simulink library "RespiratorCtrlLib"  (R2018b)
settings: Solver=VariableStepAuto  StartTime=0.0  StopTime=10.0  RelTol=1e-3
undefined symbols (not defined in the file or in its folder): AnalogMax, AnalogMin, aValveFullClose, aValveFullOpen, aValvePwm100, eSupervisorStates, fpDiffQAirInhalation, fpStatQAirInhalation, pDiffQAirAutoOffsetMax, pDiffQAirAutoOffsetMin, pDiffQAirAutoOffsetRateMax, pDiffQAirInhalationOffset, pDiffQAirScaledMax, pDiffQAirScaledMin, PressureMax, PressureMin, pStatQAirAutoOffsetMax, pStatQAirAutoOffsetMin, pStatQAirAutoOffsetRateMax, pStatQAirInhalationOffset, pStatQAirScaledMax, pStatQAirScaledMin, rPwmZeroDeg, VAnalogInputSpan, VpDiffQAirAnalogicDiagMax, VpDiffQAirAnalogicDiagMin, VpDiffQAirAnalogicMax, VpDiffQAirAnalogicMin, VpStatQAirAnalogicDiagMax, VpStatQAirAnalogicDiagMin, VpStatQAirAnalogicMax, VpStatQAirAnalogicMin
libraries: simulink x16, mbedblockslib x4, simulink_extras x2, $bdroot x2
(part 2 of 2)

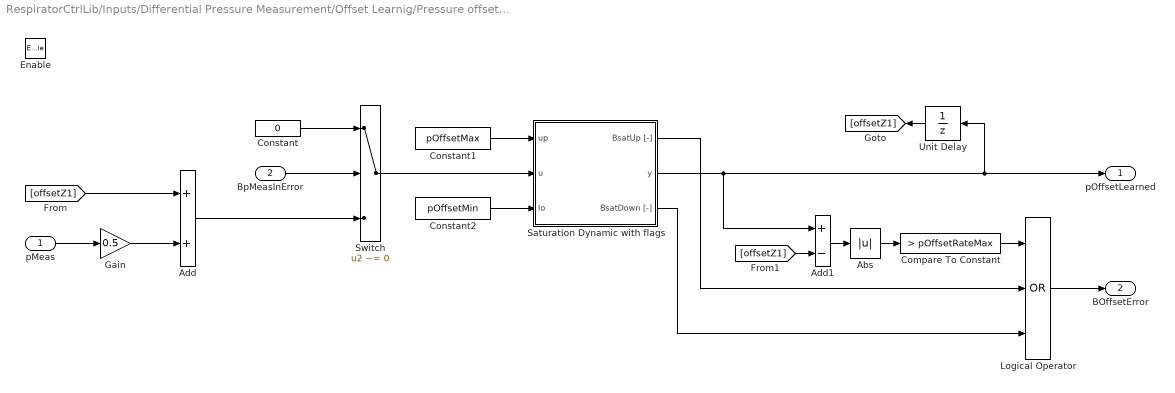
== system RespiratorCtrlLib/Inputs/Differential Pressure Measurement/Offset Learnig/Pressure offset computation ==
  pMeas : Inport
  BpMeasInError : Inport  Port=2
  Enable : EnablePort  StatesWhenEnabling=reset
  Abs : Abs
  Add : Sum
  Add1 : Sum  Inputs=+-
  Compare To Constant : simulink/Logic and Bit Operations/Compare To Constant  relop=>  const=pOffsetRateMax  OutDataTypeStr=boolean
  Constant : Constant  Value=0  OutDataTypeStr=single
  Constant1 : Constant  Value=pOffsetMax  OutDataTypeStr=single
  Constant2 : Constant  Value=pOffsetMin  OutDataTypeStr=single
  Gain : Gain  Gain=0.5
  Logical Operator : Logic  Operator=OR  Inputs=3  AllPortsSameDT=off  OutDataTypeStr=boolean
  Saturation Dynamic with flags : Subsystem  mask(Saturation Dynamic){OutMin=[], OutMax=[], OutDataTypeStr=Inherit: Same as second input, OutputDataTypeScalingMode=Same as second input, OutDataType=fixdt(1, 16), OutScaling=2^-10, LockScale=off, RndMeth=Floor, DoSatur=off}
      mask prompts: OutMin "Output minimum:"; OutMax "Output maximum:"; OutDataTypeStr "Output data type:"; OutputDataTypeScalingMode "Output data type mode:"; OutDataType "Output data type (e.g. fixdt(1, 16), fixdt('single')):"; OutScaling "Output scaling (Slope, e.g. 2^-9 or [Slope Bias], e.g. [1.25 3]):"; LockScale "Lock output data type setting against changes by the fixed-point tools"; RndMeth "Integer rounding mode:"; DoSatur "Saturate on integer overflow"
      mask help: Bound the range of the second input by using the first input (upper limit) and the third input (lower limit).
      mask init: same as RespiratorCtrlLib/Inputs/Static Pressures Offset/Pressure offset computation/Saturation Dynamic with flags
      mask Callback OutDataTypeStr: fixptdialog(gcbh)
      mask TypeOptions OutputDataTypeScalingMode: double | single | int8 | uint8 | int16 | uint16 | int32 | uint32 | Specify via dialog | Same as second input
      mask Callback OutputDataTypeScalingMode: fixptdialog(gcbh)
      mask Callback OutDataType: fixptdialog(gcbh)
      mask TypeOptions RndMeth: Ceiling | Convergent | Floor | Nearest | Round | Simplest | Zero
      mask Display: plot([0.15 0.85],[.5 .5],[.5 .5],[0.05 0.95],0.15+0.7*[0 .25 .75 1],0.05+0.9*[.25 .25 .75 .75]);
  Switch : Switch  Criteria=u2 ~= 0
  Unit Delay : UnitDelay  SampleTime=-1
  pOffsetLearned : Outport  InitialOutput=0
  BOffsetError : Outport  Port=2  OutDataTypeStr=boolean  InitialOutput=false
  wires:
  BpMeasInError/1 -> Switch/2
  Constant/1 -> Switch/1
  Unit Delay/1 -> [offsetZ1]
  pMeas/1 -> Gain/1
  Gain/1 -> Add/2
  [offsetZ1] -> Add/1
  Add/1 -> Switch/3
  Switch/1 -> Saturation Dynamic with flags/2(u)
  Saturation Dynamic with flags/2(y) -> Unit Delay/1, pOffsetLearned/1, Add1/1
  Constant1/1 -> Saturation Dynamic with flags/1(up)
  Constant2/1 -> Saturation Dynamic with flags/3(lo)
  [offsetZ1] -> Add1/2
  Add1/1 -> Abs/1
  Abs/1 -> Compare To Constant/1
  Compare To Constant/1 -> Logical Operator/1
  Saturation Dynamic with flags/1(BsatUp [-]) -> Logical Operator/2
  Saturation Dynamic with flags/3(BsatDown [-]) -> Logical Operator/3
  Logical Operator/1 -> BOffsetError/1

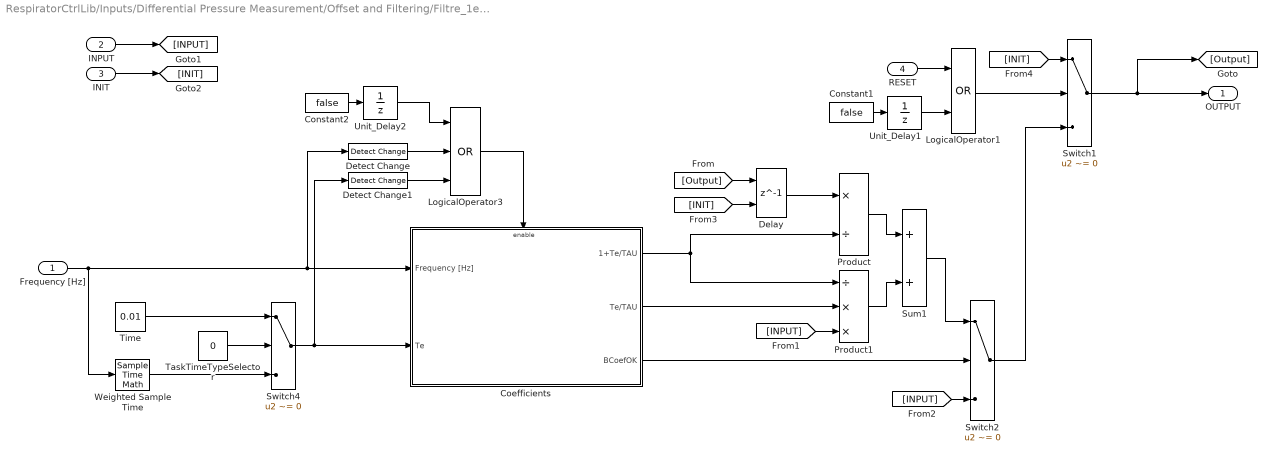
== system RespiratorCtrlLib/Inputs/Differential Pressure Measurement/Offset and Filtering/Filtre_1er_ordre_Init ==
  Frequency [Hz] : Inport  Tag=AM,In,0,1,Name,C;CMP,Port,PortWidth,SampleTime;
  INPUT : Inport  Tag=AM,In,0,1,Name,C;CMP,Port,PortWidth,SampleTime;  Port=2
  INIT : Inport  Tag=AM,In,0,1,Name,C;CMP,Port,PortWidth,SampleTime;  Port=3
  RESET : Inport  Tag=AM,In,0,1,Name,C;CMP,Port,PortWidth,SampleTime;  Port=4
  Coefficients : Subsystem
  Constant1 : Constant  Value=false
  Constant2 : Constant  Value=false
  Delay : Delay  DelayLength=1  InitialConditionSource=Input port  InitialCondition=0
      settings: InputPortMap=u0,p4
  Detect Change : simulink/Logic and Bit Operations/Detect Change  vinit=0  OutDataTypeStr=boolean
  Detect Change1 : simulink/Logic and Bit Operations/Detect Change  vinit=0  OutDataTypeStr=boolean
  LogicalOperator1 : Logic  Operator=OR  AllPortsSameDT=off  OutDataTypeStr=boolean
  LogicalOperator3 : Logic  Operator=OR  Inputs=3  AllPortsSameDT=off  OutDataTypeStr=boolean
  Product : Product  Inputs=*/  SaturateOnIntegerOverflow=on  RndMeth=Zero  InputSameDT=on  OutDataTypeStr=Inherit: Same as first input
  Product1 : Product  Inputs=/**  SaturateOnIntegerOverflow=on  RndMeth=Zero  InputSameDT=on  OutDataTypeStr=Inherit: Same as first input
  Sum1 : Sum  SaturateOnIntegerOverflow=on  InputSameDT=on  OutDataTypeStr=Inherit: Same as first input
  Switch1 : Switch  Tag=GEN,Threshold;AM,Switch,2,1;CMP,Threshold;  Criteria=u2 ~= 0  Threshold=0.5  SaturateOnIntegerOverflow=on  InputSameDT=on
  Switch2 : Switch  Tag=GEN,Threshold;AM,Switch,2,1;CMP,Threshold;  Criteria=u2 ~= 0  SaturateOnIntegerOverflow=on  InputSameDT=on
  Switch4 : Switch  Tag=GEN,Threshold;AM,Switch,2,1;CMP,Threshold;  Criteria=u2 ~= 0  Threshold=0.5  SaturateOnIntegerOverflow=on  InputSameDT=on
  TaskTimeTypeSelector : Constant  Value=0  OutDataTypeStr=boolean
  Time : Constant  Value=0.01  OutDataTypeStr=Inherit: Inherit via back propagation
  Unit_Delay1 : UnitDelay  InitialCondition=true  SampleTime=-1
      settings: AttributesFormatString=IC = %<X0>
  Unit_Delay2 : UnitDelay  InitialCondition=true  SampleTime=-1
      settings: AttributesFormatString=IC = %<X0>
  Weighted Sample Time : SampleTimeMath  TsampMathOp=Ts Only  OutDataTypeStr=Inherit: Inherit via back propagation
  OUTPUT : Outport  Tag=AM,Out,1,0,Name,NC;CMP,Port,OutputWhenDisabled,InitialOutput;
  wires:
  Constant1/1 -> Unit_Delay1/1
  Unit_Delay2/1 -> LogicalOperator3/1
  Constant2/1 -> Unit_Delay2/1
  Coefficients/3(BCoefOK) -> Switch2/2
  Sum1/1 -> Switch2/1
  [INPUT] -> Switch2/3
  Detect Change1/1 -> LogicalOperator3/3
  Detect Change/1 -> LogicalOperator3/2
  LogicalOperator3/1 -> Coefficients/Enable
  TaskTimeTypeSelector/1 -> Switch4/2
  Time/1 -> Switch4/1
  Switch4/1 -> Detect Change1/1, Coefficients/2(Te)
  Weighted Sample Time/1 -> Switch4/3
  Frequency [Hz]/1 -> Weighted Sample Time/1, Detect Change/1, Coefficients/1(Frequency [Hz])
  Coefficients/2(Te/TAU) -> Product1/2
  Coefficients/1(1+Te/TAU) -> Product/2, Product1/1
  Switch2/1 -> Switch1/3
  [INIT] -> Switch1/1
  [INIT] -> Delay/2
  [INPUT] -> Product1/3
  INIT/1 -> [INIT]
  INPUT/1 -> [INPUT]
  Product/1 -> Sum1/1
  Product1/1 -> Sum1/2
  LogicalOperator1/1 -> Switch1/2
  Delay/1 -> Product/1
  Unit_Delay1/1 -> LogicalOperator1/2
  RESET/1 -> LogicalOperator1/1
  [Output] -> Delay/1
  Switch1/1 -> OUTPUT/1, [Output]

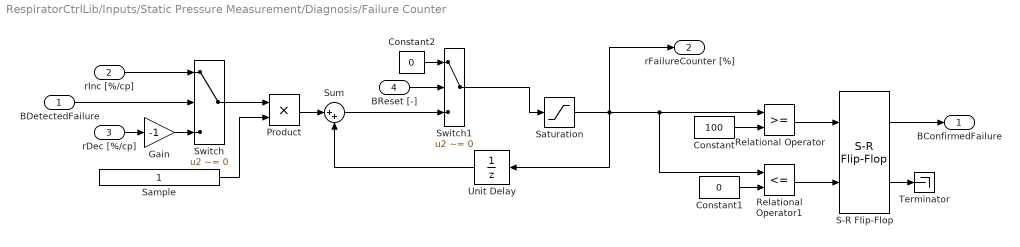
== system RespiratorCtrlLib/Inputs/Static Pressure Measurement/Diagnosis/Failure Counter ==
  BDetectedFailure : Inport
  rInc [%/cp] : Inport  Port=2
  rDec [%/cp] : Inport  Port=3
  BReset [-] : Inport  Port=4
  Constant : Constant  Value=100
  Constant1 : Constant  Value=0
  Constant2 : Constant  Value=0
  Gain : Gain  Gain=-1
  Product : Product  RndMeth=Zero
  Relational Operator : RelationalOperator  OutDataTypeStr=boolean  RndMeth=Nearest
  Relational Operator1 : RelationalOperator  Operator=<=  OutDataTypeStr=boolean  RndMeth=Nearest
  S-R Flip-Flop : simulink_extras/Flip Flops/S-R Flip-Flop  initial_condition=0
  Sample : Constant
  Saturation : Saturate  UpperLimit=100  LowerLimit=0
      settings: AttributesFormatString=[%<LowerLimit>;%<UpperLimit>]
  Sum : Sum  Inputs=|++
  Switch : Switch  Criteria=u2 ~= 0
  Switch1 : Switch  Criteria=u2 ~= 0
  Terminator : Terminator
  Unit Delay : UnitDelay  SampleTime=-1
  BConfirmedFailure : Outport
  rFailureCounter [%] : Outport  Port=2
  wires:
  Switch1/1 -> Saturation/1
  BReset [-]/1 -> Switch1/2
  Constant2/1 -> Switch1/1
  S-R Flip-Flop/2 -> Terminator/1
  BDetectedFailure/1 -> Switch/2
  rInc [%/cp]/1 -> Switch/1
  rDec [%/cp]/1 -> Gain/1
  Switch/1 -> Product/1
  Sum/1 -> Switch1/3
  S-R Flip-Flop/1 -> BConfirmedFailure/1
  Unit Delay/1 -> Sum/2
  Saturation/1 -> Unit Delay/1, rFailureCounter [%]/1, Relational Operator/1, Relational Operator1/1
  Constant/1 -> Relational Operator/2
  Relational Operator/1 -> S-R Flip-Flop/1
  Relational Operator1/1 -> S-R Flip-Flop/2
  Constant1/1 -> Relational Operator1/2
  Gain/1 -> Switch/3
  Sample/1 -> Product/2
  Product/1 -> Sum/1

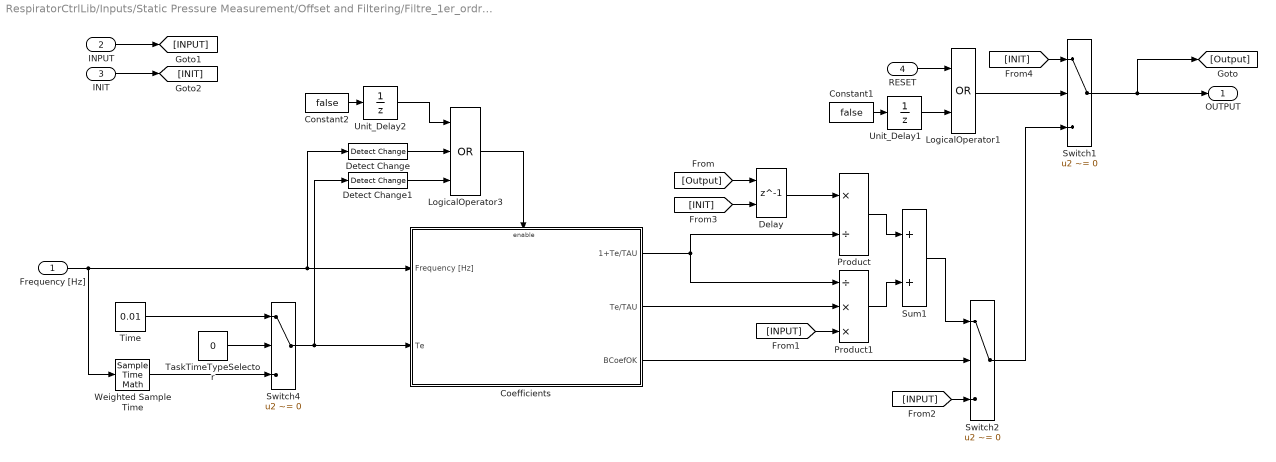
== system RespiratorCtrlLib/Inputs/Static Pressure Measurement/Offset and Filtering/Filtre_1er_ordre_Init ==
  Frequency [Hz] : Inport  Tag=AM,In,0,1,Name,C;CMP,Port,PortWidth,SampleTime;
  INPUT : Inport  Tag=AM,In,0,1,Name,C;CMP,Port,PortWidth,SampleTime;  Port=2
  INIT : Inport  Tag=AM,In,0,1,Name,C;CMP,Port,PortWidth,SampleTime;  Port=3
  RESET : Inport  Tag=AM,In,0,1,Name,C;CMP,Port,PortWidth,SampleTime;  Port=4
  Coefficients : Subsystem
  Constant1 : Constant  Value=false
  Constant2 : Constant  Value=false
  Delay : Delay  DelayLength=1  InitialConditionSource=Input port  InitialCondition=0
      settings: InputPortMap=u0,p4
  Detect Change : simulink/Logic and Bit Operations/Detect Change  vinit=0  OutDataTypeStr=boolean
  Detect Change1 : simulink/Logic and Bit Operations/Detect Change  vinit=0  OutDataTypeStr=boolean
  LogicalOperator1 : Logic  Operator=OR  AllPortsSameDT=off  OutDataTypeStr=boolean
  LogicalOperator3 : Logic  Operator=OR  Inputs=3  AllPortsSameDT=off  OutDataTypeStr=boolean
  Product : Product  Inputs=*/  SaturateOnIntegerOverflow=on  RndMeth=Zero  InputSameDT=on  OutDataTypeStr=Inherit: Same as first input
  Product1 : Product  Inputs=/**  SaturateOnIntegerOverflow=on  RndMeth=Zero  InputSameDT=on  OutDataTypeStr=Inherit: Same as first input
  Sum1 : Sum  SaturateOnIntegerOverflow=on  InputSameDT=on  OutDataTypeStr=Inherit: Same as first input
  Switch1 : Switch  Tag=GEN,Threshold;AM,Switch,2,1;CMP,Threshold;  Criteria=u2 ~= 0  Threshold=0.5  SaturateOnIntegerOverflow=on  InputSameDT=on
  Switch2 : Switch  Tag=GEN,Threshold;AM,Switch,2,1;CMP,Threshold;  Criteria=u2 ~= 0  SaturateOnIntegerOverflow=on  InputSameDT=on
  Switch4 : Switch  Tag=GEN,Threshold;AM,Switch,2,1;CMP,Threshold;  Criteria=u2 ~= 0  Threshold=0.5  SaturateOnIntegerOverflow=on  InputSameDT=on
  TaskTimeTypeSelector : Constant  Value=0  OutDataTypeStr=boolean
  Time : Constant  Value=0.01  OutDataTypeStr=Inherit: Inherit via back propagation
  Unit_Delay1 : UnitDelay  InitialCondition=true  SampleTime=-1
      settings: AttributesFormatString=IC = %<X0>
  Unit_Delay2 : UnitDelay  InitialCondition=true  SampleTime=-1
      settings: AttributesFormatString=IC = %<X0>
  Weighted Sample Time : SampleTimeMath  TsampMathOp=Ts Only  OutDataTypeStr=Inherit: Inherit via back propagation
  OUTPUT : Outport  Tag=AM,Out,1,0,Name,NC;CMP,Port,OutputWhenDisabled,InitialOutput;
  wires:
  Switch1/1 -> [Output], OUTPUT/1
  [Output] -> Delay/1
  RESET/1 -> LogicalOperator1/1
  Unit_Delay1/1 -> LogicalOperator1/2
  Delay/1 -> Product/1
  LogicalOperator1/1 -> Switch1/2
  Product1/1 -> Sum1/2
  Product/1 -> Sum1/1
  INPUT/1 -> [INPUT]
  INIT/1 -> [INIT]
  [INPUT] -> Product1/3
  [INIT] -> Delay/2
  [INIT] -> Switch1/1
  Switch2/1 -> Switch1/3
  Coefficients/1(1+Te/TAU) -> Product1/1, Product/2
  Coefficients/2(Te/TAU) -> Product1/2
  Frequency [Hz]/1 -> Coefficients/1(Frequency [Hz]), Detect Change/1, Weighted Sample Time/1
  Weighted Sample Time/1 -> Switch4/3
  Switch4/1 -> Coefficients/2(Te), Detect Change1/1
  Time/1 -> Switch4/1
  TaskTimeTypeSelector/1 -> Switch4/2
  LogicalOperator3/1 -> Coefficients/Enable
  Detect Change/1 -> LogicalOperator3/2
  Detect Change1/1 -> LogicalOperator3/3
  [INPUT] -> Switch2/3
  Sum1/1 -> Switch2/1
  Coefficients/3(BCoefOK) -> Switch2/2
  Constant2/1 -> Unit_Delay2/1
  Unit_Delay2/1 -> LogicalOperator3/1
  Constant1/1 -> Unit_Delay1/1

== system RespiratorCtrlLib/Inputs/Static Pressures Offset/Pressure offset computation/Saturation Dynamic with flags ==
  up : Inport
  u : Inport  Port=2
  lo : Inport  Port=3
  Data Type Duplicate : DataTypeDuplicate
  Data Type Propagation : simulink/Signal Attributes/Data Type Propagation  PropDataType=fixdt(1, 16)  IfRefDouble=double  IfRefSingle=single  IsSigned=IsSigned1  NumBitsBase=NumBits1  NumBitsMult=1  NumBitsAdd=0  NumBitsAllowFinal=1:128  PropScaling=2^-10  ValuesUsedBestPrec=[5 -7]  SlopeBase=Slope1  SlopeMult=1  SlopeAdd=0  BiasBase=Bias1  BiasMult=1  BiasAdd=0
      settings: SourceProductName=Simulink  SourceProductBaseCode=SL
  LowerRelop1 : RelationalOperator  DisableCoverage=on  Operator=>  OutDataTypeStr=boolean  RndMeth=Nearest
  Switch : Switch  Criteria=u2 ~= 0  OutDataTypeStr=Inherit: Inherit via back propagation  ZeroCross=off
  Switch2 : Switch  Criteria=u2 ~= 0  OutMin=OutMin  OutMax=OutMax  OutDataTypeStr=Inherit: Inherit via back propagation  ZeroCross=off
  UpperRelop : RelationalOperator  DisableCoverage=on  Operator=<  OutDataTypeStr=boolean  RndMeth=Nearest
  BsatUp [-] : Outport  OutMin=OutMin  OutMax=OutMax
  y : Outport  Port=2  OutMin=OutMin  OutMax=OutMax
  BsatDown [-] : Outport  Port=3  OutMin=OutMin  OutMax=OutMax
  wires:
  up/1 -> Switch2/1, LowerRelop1/2
  u/1 -> Data Type Propagation/2, Data Type Propagation/1, LowerRelop1/1, Switch/3, UpperRelop/1
  lo/1 -> Switch/1, UpperRelop/2
  Switch/1 -> Data Type Duplicate/2, Switch2/3, Data Type Propagation/3
  Switch2/1 -> Data Type Duplicate/1, y/1
  LowerRelop1/1 -> Switch2/2, BsatUp [-]/1
  UpperRelop/1 -> BsatDown [-]/1, Switch/2

== system RespiratorCtrlLib/Inputs/Differential Pressure Measurement/Offset Learnig/Pressure offset computation/Saturation Dynamic with flags ==
  up : Inport
  u : Inport  Port=2
  lo : Inport  Port=3
  Data Type Duplicate : DataTypeDuplicate
  Data Type Propagation : simulink/Signal Attributes/Data Type Propagation  PropDataType=fixdt(1, 16)  IfRefDouble=double  IfRefSingle=single  IsSigned=IsSigned1  NumBitsBase=NumBits1  NumBitsMult=1  NumBitsAdd=0  NumBitsAllowFinal=1:128  PropScaling=2^-10  ValuesUsedBestPrec=[5 -7]  SlopeBase=Slope1  SlopeMult=1  SlopeAdd=0  BiasBase=Bias1  BiasMult=1  BiasAdd=0
      settings: SourceProductName=Simulink  SourceProductBaseCode=SL
  LowerRelop1 : RelationalOperator  DisableCoverage=on  Operator=>  OutDataTypeStr=boolean  RndMeth=Nearest
  Switch : Switch  Criteria=u2 ~= 0  OutDataTypeStr=Inherit: Inherit via back propagation  ZeroCross=off
  Switch2 : Switch  Criteria=u2 ~= 0  OutMin=OutMin  OutMax=OutMax  OutDataTypeStr=Inherit: Inherit via back propagation  ZeroCross=off
  UpperRelop : RelationalOperator  DisableCoverage=on  Operator=<  OutDataTypeStr=boolean  RndMeth=Nearest
  BsatUp [-] : Outport  OutMin=OutMin  OutMax=OutMax
  y : Outport  Port=2  OutMin=OutMin  OutMax=OutMax
  BsatDown [-] : Outport  Port=3  OutMin=OutMin  OutMax=OutMax
  wires:
  up/1 -> Switch2/1, LowerRelop1/2
  u/1 -> Data Type Propagation/2, Data Type Propagation/1, LowerRelop1/1, Switch/3, UpperRelop/1
  lo/1 -> Switch/1, UpperRelop/2
  Switch/1 -> Data Type Duplicate/2, Switch2/3, Data Type Propagation/3
  Switch2/1 -> Data Type Duplicate/1, y/1
  LowerRelop1/1 -> Switch2/2, BsatUp [-]/1
  UpperRelop/1 -> BsatDown [-]/1, Switch/2

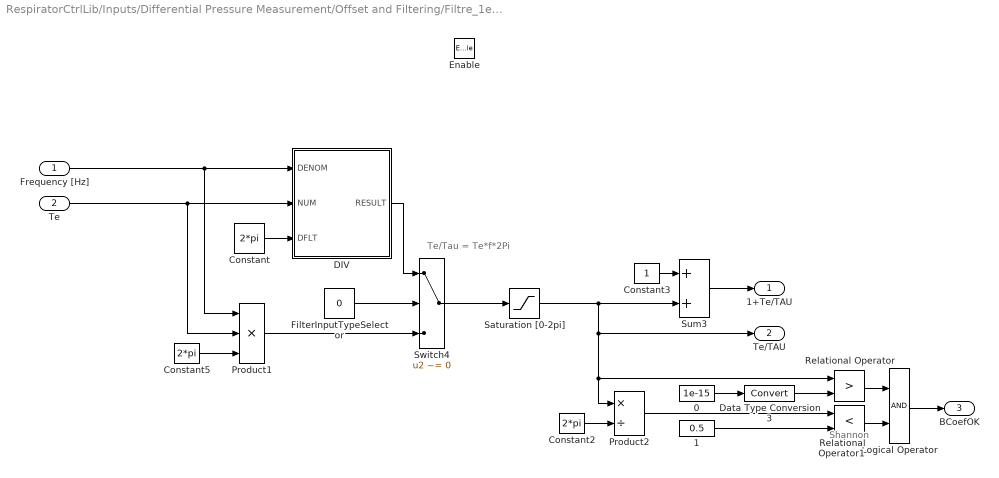
== system RespiratorCtrlLib/Inputs/Differential Pressure Measurement/Offset and Filtering/Filtre_1er_ordre_Init/Coefficients ==
  note: Te/Tau = Te*f*2Pi
  note: Shannon
  Frequency [Hz] : Inport
  Te : Inport  Port=2
  Enable : EnablePort
  0 : Constant  Value=1e-15  OutDataTypeStr=Inherit: Inherit via back propagation
  1 : Constant  Value=0.5  OutDataTypeStr=Inherit: Inherit via back propagation
  Constant : Constant  Value=2*pi  OutDataTypeStr=Inherit: Inherit via back propagation
  Constant2 : Constant  Value=2*pi  OutDataTypeStr=Inherit: Inherit via back propagation
  Constant3 : Constant  OutDataTypeStr=Inherit: Inherit via back propagation
  Constant5 : Constant  Value=2*pi  OutDataTypeStr=Inherit: Inherit via back propagation
  DIV : Subsystem  mask(DIV){}
      mask help: This block executes a division with protection for division by 0.
      mask Display: disp('DIV')
  Data Type Conversion3 : DataTypeConversion
  FilterInputTypeSelector : Constant  Value=0  OutDataTypeStr=boolean
  Logical Operator : Logic  AllPortsSameDT=off
  Product1 : Product  Inputs=***  SaturateOnIntegerOverflow=on  RndMeth=Zero  InputSameDT=on  OutDataTypeStr=Inherit: Same as first input
  Product2 : Product  Inputs=*/  SaturateOnIntegerOverflow=on  RndMeth=Zero  InputSameDT=on  OutDataTypeStr=Inherit: Same as first input
  Relational Operator : RelationalOperator  Operator=>  RndMeth=Nearest  InputSameDT=on
  Relational Operator1 : RelationalOperator  Operator=<  RndMeth=Nearest  InputSameDT=on
  Saturation [0-2pi] : Saturate  UpperLimit=2*pi  LowerLimit=0  OutDataTypeStr=Inherit: Inherit via back propagation
  Sum3 : Sum  OutDataTypeStr=Inherit: Inherit via back propagation  RndMeth=Zero  InputSameDT=on
  Switch4 : Switch  Tag=GEN,Threshold;AM,Switch,2,1;CMP,Threshold;  Criteria=u2 ~= 0  Threshold=0.5  SaturateOnIntegerOverflow=on  InputSameDT=on
  1+Te/TAU : Outport
  Te/TAU : Outport  Port=2
  BCoefOK : Outport  Port=3
  wires:
  Logical Operator/1 -> BCoefOK/1
  Data Type Conversion3/1 -> Relational Operator/2
  0/1 -> Data Type Conversion3/1
  Saturation [0-2pi]/1 -> Sum3/2, Relational Operator/1, Product2/1, Te/TAU/1
  1/1 -> Relational Operator1/2
  Relational Operator/1 -> Logical Operator/1
  Relational Operator1/1 -> Logical Operator/2
  Product2/1 -> Relational Operator1/1
  FilterInputTypeSelector/1 -> Switch4/2
  Switch4/1 -> Saturation [0-2pi]/1
  Product1/1 -> Switch4/3
  DIV/1(RESULT) -> Switch4/1
  Constant5/1 -> Product1/3
  Te/1 -> DIV/2(NUM), Product1/2
  Frequency [Hz]/1 -> DIV/1(DENOM), Product1/1
  Constant2/1 -> Product2/2
  Constant3/1 -> Sum3/1
  Sum3/1 -> 1+Te/TAU/1
  Constant/1 -> DIV/3(DFLT)

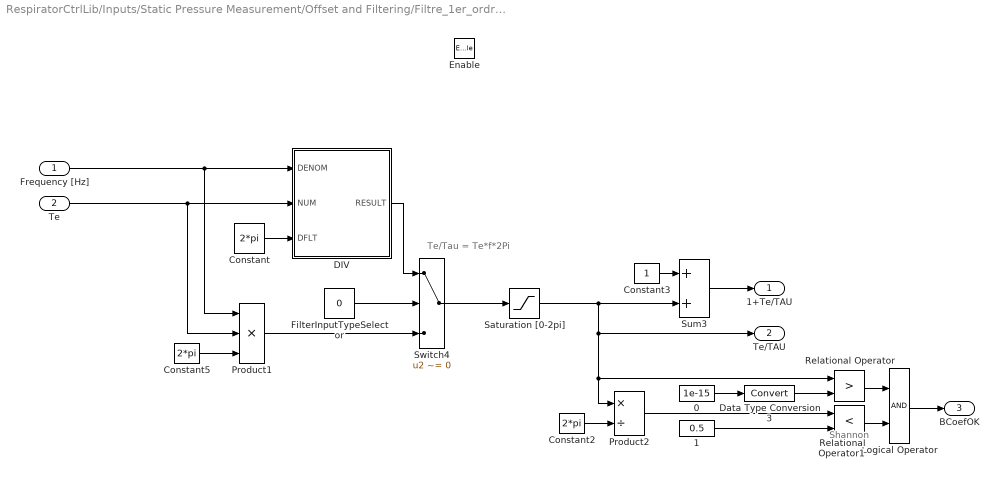
== system RespiratorCtrlLib/Inputs/Static Pressure Measurement/Offset and Filtering/Filtre_1er_ordre_Init/Coefficients ==
  note: Shannon
  note: Te/Tau = Te*f*2Pi
  Frequency [Hz] : Inport
  Te : Inport  Port=2
  Enable : EnablePort
  0 : Constant  Value=1e-15  OutDataTypeStr=Inherit: Inherit via back propagation
  1 : Constant  Value=0.5  OutDataTypeStr=Inherit: Inherit via back propagation
  Constant : Constant  Value=2*pi  OutDataTypeStr=Inherit: Inherit via back propagation
  Constant2 : Constant  Value=2*pi  OutDataTypeStr=Inherit: Inherit via back propagation
  Constant3 : Constant  OutDataTypeStr=Inherit: Inherit via back propagation
  Constant5 : Constant  Value=2*pi  OutDataTypeStr=Inherit: Inherit via back propagation
  DIV : Subsystem  mask(DIV){}
      mask help: This block executes a division with protection for division by 0.
      mask Display: disp('DIV')
  Data Type Conversion3 : DataTypeConversion
  FilterInputTypeSelector : Constant  Value=0  OutDataTypeStr=boolean
  Logical Operator : Logic  AllPortsSameDT=off
  Product1 : Product  Inputs=***  SaturateOnIntegerOverflow=on  RndMeth=Zero  InputSameDT=on  OutDataTypeStr=Inherit: Same as first input
  Product2 : Product  Inputs=*/  SaturateOnIntegerOverflow=on  RndMeth=Zero  InputSameDT=on  OutDataTypeStr=Inherit: Same as first input
  Relational Operator : RelationalOperator  Operator=>  RndMeth=Nearest  InputSameDT=on
  Relational Operator1 : RelationalOperator  Operator=<  RndMeth=Nearest  InputSameDT=on
  Saturation [0-2pi] : Saturate  UpperLimit=2*pi  LowerLimit=0  OutDataTypeStr=Inherit: Inherit via back propagation
  Sum3 : Sum  OutDataTypeStr=Inherit: Inherit via back propagation  RndMeth=Zero  InputSameDT=on
  Switch4 : Switch  Tag=GEN,Threshold;AM,Switch,2,1;CMP,Threshold;  Criteria=u2 ~= 0  Threshold=0.5  SaturateOnIntegerOverflow=on  InputSameDT=on
  1+Te/TAU : Outport
  Te/TAU : Outport  Port=2
  BCoefOK : Outport  Port=3
  wires:
  Constant/1 -> DIV/3(DFLT)
  Sum3/1 -> 1+Te/TAU/1
  Constant3/1 -> Sum3/1
  Constant2/1 -> Product2/2
  Frequency [Hz]/1 -> Product1/1, DIV/1(DENOM)
  Te/1 -> Product1/2, DIV/2(NUM)
  Constant5/1 -> Product1/3
  DIV/1(RESULT) -> Switch4/1
  Product1/1 -> Switch4/3
  Switch4/1 -> Saturation [0-2pi]/1
  FilterInputTypeSelector/1 -> Switch4/2
  Product2/1 -> Relational Operator1/1
  Relational Operator1/1 -> Logical Operator/2
  Relational Operator/1 -> Logical Operator/1
  1/1 -> Relational Operator1/2
  Saturation [0-2pi]/1 -> Te/TAU/1, Product2/1, Relational Operator/1, Sum3/2
  0/1 -> Data Type Conversion3/1
  Data Type Conversion3/1 -> Relational Operator/2
  Logical Operator/1 -> BCoefOK/1

== system RespiratorCtrlLib/Inputs/Differential Pressure Measurement/Offset and Filtering/Filtre_1er_ordre_Init/Coefficients/DIV ==
  DENOM : Inport
  NUM : Inport  Port=2
  DFLT : Inport  Port=3
  Action_Else : Subsystem  TreatAsAtomicUnit=on
  Action_If : Subsystem  TreatAsAtomicUnit=on
  If : If  IfExpression=u1 ~= 0
  Merge : Merge
  RESULT : Outport
  wires:
  If/1 -> Action_If/Action
  NUM/1 -> Action_If/1(NUM)
  DENOM/1 -> Action_If/2(DENOM), If/1
  DFLT/1 -> Action_Else/1(DFLT)
  If/2 -> Action_Else/Action
  Action_If/1(RESULT) -> Merge/1
  Action_Else/1(RESULT) -> Merge/2
  Merge/1 -> RESULT/1

== system RespiratorCtrlLib/Inputs/Static Pressure Measurement/Offset and Filtering/Filtre_1er_ordre_Init/Coefficients/DIV ==
  DENOM : Inport
  NUM : Inport  Port=2
  DFLT : Inport  Port=3
  Action_Else : Subsystem  TreatAsAtomicUnit=on
  Action_If : Subsystem  TreatAsAtomicUnit=on
  If : If  IfExpression=u1 ~= 0
  Merge : Merge
  RESULT : Outport
  wires:
  Merge/1 -> RESULT/1
  Action_Else/1(RESULT) -> Merge/2
  Action_If/1(RESULT) -> Merge/1
  If/2 -> Action_Else/Action
  DFLT/1 -> Action_Else/1(DFLT)
  DENOM/1 -> If/1, Action_If/2(DENOM)
  NUM/1 -> Action_If/1(NUM)
  If/1 -> Action_If/Action

== system RespiratorCtrlLib/Inputs/Differential Pressure Measurement/Offset and Filtering/Filtre_1er_ordre_Init/Coefficients/DIV/Action_Else ==
  DFLT : Inport
  Action Port : ActionPort
  Signal Conversion : SignalConversion  OverrideOpt=off
  RESULT : Outport
  wires:
  DFLT/1 -> Signal Conversion/1
  Signal Conversion/1 -> RESULT/1

== system RespiratorCtrlLib/Inputs/Differential Pressure Measurement/Offset and Filtering/Filtre_1er_ordre_Init/Coefficients/DIV/Action_If ==
  NUM : Inport
  DENOM : Inport  Port=2
  Action Port : ActionPort
  Ideal gas law2 : Product  Inputs=*/
  RESULT : Outport
  wires:
  NUM/1 -> Ideal gas law2/1
  Ideal gas law2/1 -> RESULT/1
  DENOM/1 -> Ideal gas law2/2

== system RespiratorCtrlLib/Inputs/Static Pressure Measurement/Offset and Filtering/Filtre_1er_ordre_Init/Coefficients/DIV/Action_Else ==
  DFLT : Inport
  Action Port : ActionPort
  Signal Conversion : SignalConversion  OverrideOpt=off
  RESULT : Outport
  wires:
  Signal Conversion/1 -> RESULT/1
  DFLT/1 -> Signal Conversion/1

== system RespiratorCtrlLib/Inputs/Static Pressure Measurement/Offset and Filtering/Filtre_1er_ordre_Init/Coefficients/DIV/Action_If ==
  NUM : Inport
  DENOM : Inport  Port=2
  Action Port : ActionPort
  Ideal gas law2 : Product  Inputs=*/
  RESULT : Outport
  wires:
  DENOM/1 -> Ideal gas law2/2
  Ideal gas law2/1 -> RESULT/1
  NUM/1 -> Ideal gas law2/1

== stateflow chart RespiratorCtrlLib/Inputs/Button Processing/Push button debouce FSM ==
  state Released
    entry:
    BtnPressed = false;
    Released -> (junction 7) [order 1]
    (junction 7) -> (junction 9) [order 1] : [BtnIn == true]
    (junction 9) -> (junction 28) [order 1] : [Cnt < 65535]
    (junction 7) -> (junction 70) [order 2]
    (junction 9) -> (junction 12) [order 2]
    (junction 28) -> (junction 29) : {Cnt = Cnt + 1;}
    (junction 70) -> (junction 72) [order 1] : [Cnt > 0]
    (junction 70) -> (junction 66) [order 2]
    (junction 72) -> (junction 74) : {Cnt = Cnt - 1;}
    (junction 74) -> (junction 66)
    (junction 12) -> (junction 74)
    (junction 29) -> (junction 12)
  state Pressed
    entry:
    BtnPressed = true;
    Pressed -> (junction 94) [order 1]
    (junction 94) -> (junction 97) [order 1] : [BtnIn == true]
    (junction 97) -> (junction 95) [order 1] : [Cnt < DebounceThd]
    (junction 94) -> (junction 83) [order 2]
    (junction 97) -> (junction 89) [order 2]
    (junction 95) -> (junction 88) : {Cnt = Cnt + 1;}
    (junction 83) -> (junction 82) [order 1] : [Cnt > 0]
    (junction 83) -> (junction 80) [order 2]
    (junction 82) -> (junction 79) : {Cnt = Cnt - 1;}
    (junction 79) -> (junction 80)
    (junction 89) -> (junction 79)
    (junction 88) -> (junction 89)
  (default) -> Released
  Released -> Pressed [order 1] : [Cnt >= DebounceThd]
  Pressed -> Released [order 1] : [Cnt == 0]
  data: BtnIn input boolean; BtnPressed output boolean =false; DebounceThd input uint16; Cnt local uint16 =uint16(0)
